simulink model "IPT_FCM_test"  (Simulink 7.4)
settings: Solver=ode3  StartTime=0.0  StopTime=inf  FixedStep=0.01  RelTol=1e-3
settings Model: Creator=zhaoxiangri  LastModifiedBy=sunsijun
settings DataIOCC: SaveFormat=StructureWithTime

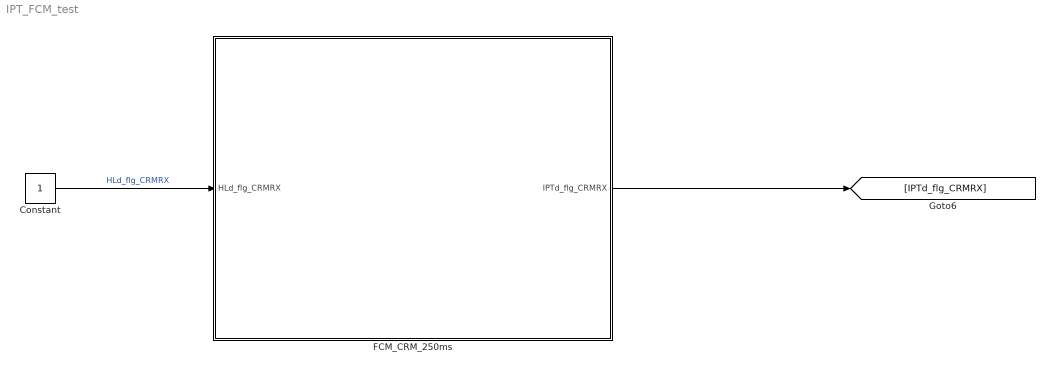
== system IPT_FCM_test ==
  Constant : Constant  OutDataTypeMode=boolean  OutDataType=fixdt(1, 16)  OutScaling=2^0  OutDataTypeStr=boolean
  FCM_CRM_250ms : Subsystem
      settings: RTWFcnNameOpts=Use subsystem name  RTWFileNameOpts=Use subsystem name
  wires:
  Constant/1 -> FCM_CRM_250ms/1(HLd_flg_CRMRX)  "HLd_flg_CRMRX"
  FCM_CRM_250ms/1(IPTd_flg_CRMRX) -> [IPTd_flg_CRMRX]

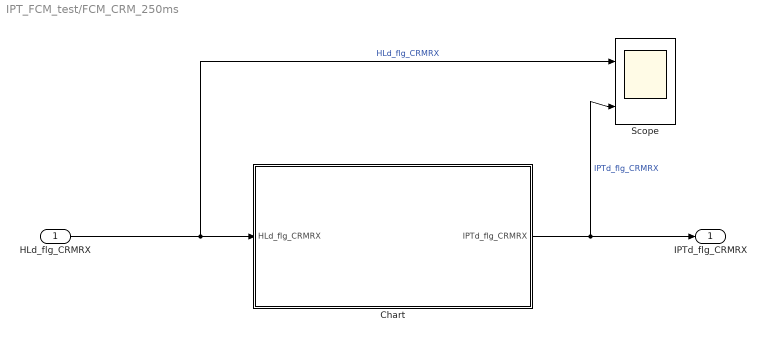
== system IPT_FCM_test/FCM_CRM_250ms ==
  HLd_flg_CRMRX : Inport
  Chart : Stateflow chart
  Scope : Scope  NumInputPorts=2
      settings: YMin=-5~-5  YMax=5~5
  IPTd_flg_CRMRX : Outport
  wires:
  Chart/1(IPTd_flg_CRMRX) -> IPTd_flg_CRMRX/1, Scope/2  "IPTd_flg_CRMRX"
  HLd_flg_CRMRX/1 -> Chart/1(HLd_flg_CRMRX), Scope/1  "HLd_flg_CRMRX"

== stateflow chart FCM_CRM_250ms/Chart ==
  state De
    (junction 4) -> (junction 5) : {IPTd_flg_CRMRX=0;}
    (default) -> (junction 4) : {IPTd_flg_CRMRX=HLd_flg_CRMRX;}
    De -> (junction 4)
  (default) -> De
  data: HLd_flg_CRMRX input boolean; IPTd_flg_CRMRX output boolean
